simulink model "ScriptDemo"  (R2022b)
settings: configuration reference "TmVcThermal_Configuration_sub" (kept outside this file)
undefined symbols (not defined in the file): aaaa, bbbb, cTmComprCtrl_D_u8HvacFlowTable_db, cTmComprCtrl_D_u8HvacFlowTable_sw, cTmComprCtrl_n_i16ChillCmpIMax, cTmComprCtrl_n_i16ChillCmpIMin, cTmComprCtrl_n_i16ChillCmpIMin666, cTmComprCtrl_n_i16ChillCmpPMax, cTmComprCtrl_n_i16ChillCmpPMin, cTmComprCtrl_n_i16CmpChillCoolRpmKiMax, cTmComprCtrl_n_i16CmpChillCoolRpmKiMin, cTmComprCtrl_n_i16CmpChillCoolRpmKpMax, cTmComprCtrl_n_i16CmpChillCoolRpmKpMin, cTmComprCtrl_n_i16CmpCoolRpmKiMax, cTmComprCtrl_n_i16CmpCoolRpmKiMin, cTmComprCtrl_n_i16CmpCoolRpmKpMax, cTmComprCtrl_n_i16CmpCoolRpmKpMin, cTmComprCtrl_n_i16SM4CmpHeatKiMax, cTmComprCtrl_n_i16SM4CmpHeatKiMin, cTmComprCtrl_n_i16SM4CmpHeatKpMax, cTmComprCtrl_n_i16SM4CmpHeatKpMin, cTmComprCtrl_n_i16SM5CmpHeatKiMax, cTmComprCtrl_n_i16SM5CmpHeatKiMin, cTmComprCtrl_n_i16SM5CmpHeatKpMax, cTmComprCtrl_n_i16SM5CmpHeatKpMin, cTmComprCtrl_n_i16SM6CmpHeatKiMax, cTmComprCtrl_n_i16SM6CmpHeatKiMin, cTmComprCtrl_n_i16SM6CmpHeatKpMax, cTmComprCtrl_n_i16SM6CmpHeatKpMin, cTmComprCtrl_n_u16CmpMaxSpdFanFltLimt, cTmComprCtrl_n_u16CmpMaxSpdLoSidePFltLimt, cTmComprCtrl_n_u16CmpMaxSpdSensorFltLimt, cTmComprCtrl_n_u16CompMinRpm, cTmComprCtrl_n_u16CompRpmIncThres, cTmComprCtrl_t_u16BattCooltFFPeriod, cTmComprCtrl_t_u16BattCooltPIPeriod, cTmComprCtrl_t_u16CmpCoolFFPeriod, cTmComprCtrl_t_u16CmpCoolPIPeriod, cTmComprCtrl_t_u16CoolCmpChillFFPeriod, cTmComprCtrl_t_u16CoolCmpChillPIPeriod, cTmComprCtrl_t_u16SM4CmpHeatFFPeriod, cTmComprCtrl_t_u16SM4CmpHeatPIPeriod, cTmComprCtrl_t_u16SM5CmpHeatFFPeriod, cTmComprCtrl_t_u16SM5CmpHeatPIPeriod, cTmComprCtrl_t_u16SM6CmpHeatFFPeriod, cTmComprCtrl_t_u16SM6CmpHeatPIPeriod, cTmComprCtrl_Te_EvapClearInteg, cTmComprCtrl_Te_i16HpReqTempSaturoffset, cTmComprCtrl_Te_i16SatLpReplaceDiff, cTmComprCtrl_Te_i16SM3BatDiffStartEvapDecOffset, cTmComprCtrl_Te_i16SM3EvapLo, cTmComprCtrl_Te_i16SM3TBatDiffEntEvapDecOffset, cTmComprCtrl_Te_i16SM3TBatDiffEntEvapDecOffsetQuit, cTmComprCtrl_Te_s32ErrCmpChillPIContinueCoolH, cTmComprCtrl_Te_s32ErrCmpChillPIContinueCoolL, cTmComprCtrl_Te_s32ErrCmpPIContinueChillH, cTmComprCtrl_Te_s32ErrCmpPIContinueChillL, cTmComprCtrl_Te_s32ErrCmpPIContinueCoolH, cTmComprCtrl_Te_s32ErrCmpPIContinueCoolL, cTmComprCtrl_Te_s32ErrCmpPIContinueHeatH ... (+398)
libraries: simulink x782, PCMULib x640, simulink_need_slupdate x4
(part 33 of 41)

== system ScriptDemo/Create/createMerge/After/SM4/ID26297_SM4FF/Flow2Rpm/Subsystem4 ==
  In1 : Inport  OutDataTypeStr=int16
  Abs : Abs  OutDataTypeStr=uint16  SaturateOnIntegerOverflow=off
  Add6 : Sum  Inputs=+-  OutDataTypeStr=int16
  Compare To Constant : simulink/Logic and Bit Operations/Compare To Constant  relop=>=  const=0  OutDataTypeStr=boolean
  Compare To Constant1 : simulink/Logic and Bit Operations/Compare To Constant  relop=<=  const=10  OutDataTypeStr=boolean
  Constant6 : Constant  Value=0  OutDataTypeStr=uint16
  Constant7 : Constant  Value=10  OutDataTypeStr=uint16
  Logical Operator : Logic  AllPortsSameDT=off  OutDataTypeStr=boolean
  Switch : Switch  Criteria=u2 ~= 0  SaturateOnIntegerOverflow=off  InputSameDT=off
  Out1 : Outport
  wires:
  Add6/1 -> Switch/1
  Logical Operator/1 -> Switch/2
  Constant6/1 -> Switch/3
  Abs/1 -> Add6/2, Compare To Constant/1, Compare To Constant1/1
  Constant7/1 -> Add6/1
  Switch/1 -> Out1/1
  Compare To Constant1/1 -> Logical Operator/2
  Compare To Constant/1 -> Logical Operator/1
  In1/1 -> Abs/1

== system ScriptDemo/Create/createMerge/After/SM4/ID26297_SM4FF/Flow2Rpm/Subsystem5 ==
  In1 : Inport  OutDataTypeStr=int16
  Abs : Abs  OutDataTypeStr=uint16  SaturateOnIntegerOverflow=off
  Add6 : Sum  Inputs=+-  OutDataTypeStr=int16
  Compare To Constant : simulink/Logic and Bit Operations/Compare To Constant  relop=>=  const=0  OutDataTypeStr=boolean
  Compare To Constant1 : simulink/Logic and Bit Operations/Compare To Constant  relop=<=  const=10  OutDataTypeStr=boolean
  Constant6 : Constant  Value=0  OutDataTypeStr=uint16
  Constant7 : Constant  Value=10  OutDataTypeStr=uint16
  Logical Operator : Logic  AllPortsSameDT=off  OutDataTypeStr=boolean
  Switch : Switch  Criteria=u2 ~= 0  SaturateOnIntegerOverflow=off  InputSameDT=off
  Out1 : Outport
  wires:
  Add6/1 -> Switch/1
  Logical Operator/1 -> Switch/2
  Constant6/1 -> Switch/3
  Abs/1 -> Add6/2, Compare To Constant/1, Compare To Constant1/1
  Constant7/1 -> Add6/1
  Switch/1 -> Out1/1
  Compare To Constant1/1 -> Logical Operator/2
  Compare To Constant/1 -> Logical Operator/1
  In1/1 -> Abs/1

== system ScriptDemo/Create/createMerge/After/SM4/ID26297_SM4FF/Flow2Rpm/XCP ==
  md_u8Blw : Inport
  Constant1 : Constant  Value=BlwHeatLevel_db
      settings: AttributesFormatString=%<Value>
  Constant28 : Constant  Value=BlwHeatLevel_sw
      settings: AttributesFormatString=%<Value>
  Switch : Switch  Criteria=u2 ~= 0  SaturateOnIntegerOverflow=off  InputSameDT=off
  Out1 : Outport
  wires:
  md_u8Blw/1 -> Switch/3
  Switch/1 -> Out1/1
  Constant28/1 -> Switch/2
  Constant1/1 -> Switch/1

== system ScriptDemo/Create/createMerge/After/SM4/SM4_Ki/Flow2Rpm/Subsystem1 ==
  In1 : Inport  OutDataTypeStr=int16
  Abs : Abs  OutDataTypeStr=single  SaturateOnIntegerOverflow=off
  Add6 : Sum  Inputs=+-  OutDataTypeStr=int16
  Compare To Constant : simulink/Logic and Bit Operations/Compare To Constant  relop=>=  const=0  OutDataTypeStr=boolean
  Compare To Constant1 : simulink/Logic and Bit Operations/Compare To Constant  relop=<=  const=10  OutDataTypeStr=boolean
  Constant6 : Constant  Value=0  OutDataTypeStr=uint16
  Constant7 : Constant  Value=10  OutDataTypeStr=uint16
  Logical Operator : Logic  AllPortsSameDT=off  OutDataTypeStr=boolean
  Switch : Switch  Criteria=u2 ~= 0  SaturateOnIntegerOverflow=off  InputSameDT=off
  Out1 : Outport
  wires:
  Add6/1 -> Switch/1
  Logical Operator/1 -> Switch/2
  Constant6/1 -> Switch/3
  Abs/1 -> Add6/2, Compare To Constant/1, Compare To Constant1/1
  Constant7/1 -> Add6/1
  Switch/1 -> Out1/1
  Compare To Constant1/1 -> Logical Operator/2
  Compare To Constant/1 -> Logical Operator/1
  In1/1 -> Abs/1

== system ScriptDemo/Create/createMerge/After/SM4/SM4_Ki/Flow2Rpm/Subsystem2 ==
  In1 : Inport  OutDataTypeStr=int16
  Abs : Abs  OutDataTypeStr=uint16  SaturateOnIntegerOverflow=off
  Add6 : Sum  Inputs=+-  OutDataTypeStr=int16
  Compare To Constant : simulink/Logic and Bit Operations/Compare To Constant  relop=>=  const=0  OutDataTypeStr=boolean
  Compare To Constant1 : simulink/Logic and Bit Operations/Compare To Constant  relop=<=  const=10  OutDataTypeStr=boolean
  Constant6 : Constant  Value=0  OutDataTypeStr=uint16
  Constant7 : Constant  Value=10  OutDataTypeStr=uint16
  Logical Operator : Logic  AllPortsSameDT=off  OutDataTypeStr=boolean
  Switch : Switch  Criteria=u2 ~= 0  SaturateOnIntegerOverflow=off  InputSameDT=off
  Out1 : Outport
  wires:
  Add6/1 -> Switch/1
  Logical Operator/1 -> Switch/2
  Constant6/1 -> Switch/3
  Abs/1 -> Add6/2, Compare To Constant/1, Compare To Constant1/1
  Constant7/1 -> Add6/1
  Switch/1 -> Out1/1
  Compare To Constant1/1 -> Logical Operator/2
  Compare To Constant/1 -> Logical Operator/1
  In1/1 -> Abs/1

== system ScriptDemo/Create/createMerge/After/SM4/SM4_Ki/Flow2Rpm/Subsystem3 ==
  In1 : Inport  OutDataTypeStr=int16
  Abs : Abs  OutDataTypeStr=uint16  SaturateOnIntegerOverflow=off
  Add6 : Sum  Inputs=+-  OutDataTypeStr=int16
  Compare To Constant : simulink/Logic and Bit Operations/Compare To Constant  relop=>=  const=0  OutDataTypeStr=boolean
  Compare To Constant1 : simulink/Logic and Bit Operations/Compare To Constant  relop=<=  const=10  OutDataTypeStr=boolean
  Constant6 : Constant  Value=0  OutDataTypeStr=uint16
  Constant7 : Constant  Value=10  OutDataTypeStr=uint16
  Logical Operator : Logic  AllPortsSameDT=off  OutDataTypeStr=boolean
  Switch : Switch  Criteria=u2 ~= 0  SaturateOnIntegerOverflow=off  InputSameDT=off
  Out1 : Outport
  wires:
  Add6/1 -> Switch/1
  Logical Operator/1 -> Switch/2
  Constant6/1 -> Switch/3
  Abs/1 -> Add6/2, Compare To Constant/1, Compare To Constant1/1
  Constant7/1 -> Add6/1
  Switch/1 -> Out1/1
  Compare To Constant1/1 -> Logical Operator/2
  Compare To Constant/1 -> Logical Operator/1
  In1/1 -> Abs/1

== system ScriptDemo/Create/createMerge/After/SM4/SM4_Ki/Flow2Rpm/Subsystem4 ==
  In1 : Inport  OutDataTypeStr=int16
  Abs : Abs  OutDataTypeStr=uint16  SaturateOnIntegerOverflow=off
  Add6 : Sum  Inputs=+-  OutDataTypeStr=int16
  Compare To Constant : simulink/Logic and Bit Operations/Compare To Constant  relop=>=  const=0  OutDataTypeStr=boolean
  Compare To Constant1 : simulink/Logic and Bit Operations/Compare To Constant  relop=<=  const=10  OutDataTypeStr=boolean
  Constant6 : Constant  Value=0  OutDataTypeStr=uint16
  Constant7 : Constant  Value=10  OutDataTypeStr=uint16
  Logical Operator : Logic  AllPortsSameDT=off  OutDataTypeStr=boolean
  Switch : Switch  Criteria=u2 ~= 0  SaturateOnIntegerOverflow=off  InputSameDT=off
  Out1 : Outport
  wires:
  Add6/1 -> Switch/1
  Logical Operator/1 -> Switch/2
  Constant6/1 -> Switch/3
  Abs/1 -> Add6/2, Compare To Constant/1, Compare To Constant1/1
  Constant7/1 -> Add6/1
  Switch/1 -> Out1/1
  Compare To Constant1/1 -> Logical Operator/2
  Compare To Constant/1 -> Logical Operator/1
  In1/1 -> Abs/1

== system ScriptDemo/Create/createMerge/After/SM4/SM4_Ki/Flow2Rpm/Subsystem5 ==
  In1 : Inport  OutDataTypeStr=int16
  Abs : Abs  OutDataTypeStr=uint16  SaturateOnIntegerOverflow=off
  Add6 : Sum  Inputs=+-  OutDataTypeStr=int16
  Compare To Constant : simulink/Logic and Bit Operations/Compare To Constant  relop=>=  const=0  OutDataTypeStr=boolean
  Compare To Constant1 : simulink/Logic and Bit Operations/Compare To Constant  relop=<=  const=10  OutDataTypeStr=boolean
  Constant6 : Constant  Value=0  OutDataTypeStr=uint16
  Constant7 : Constant  Value=10  OutDataTypeStr=uint16
  Logical Operator : Logic  AllPortsSameDT=off  OutDataTypeStr=boolean
  Switch : Switch  Criteria=u2 ~= 0  SaturateOnIntegerOverflow=off  InputSameDT=off
  Out1 : Outport
  wires:
  Add6/1 -> Switch/1
  Logical Operator/1 -> Switch/2
  Constant6/1 -> Switch/3
  Abs/1 -> Add6/2, Compare To Constant/1, Compare To Constant1/1
  Constant7/1 -> Add6/1
  Switch/1 -> Out1/1
  Compare To Constant1/1 -> Logical Operator/2
  Compare To Constant/1 -> Logical Operator/1
  In1/1 -> Abs/1

== system ScriptDemo/Create/createMerge/After/SM4/SM4_Ki/Flow2Rpm/XCP ==
  md_u8Blw : Inport
  Constant1 : Constant  Value=BlwHeatLevel_db
      settings: AttributesFormatString=%<Value>
  Constant28 : Constant  Value=BlwHeatLevel_sw
      settings: AttributesFormatString=%<Value>
  Switch : Switch  Criteria=u2 ~= 0  SaturateOnIntegerOverflow=off  InputSameDT=off
  Out1 : Outport
  wires:
  md_u8Blw/1 -> Switch/3
  Switch/1 -> Out1/1
  Constant28/1 -> Switch/2
  Constant1/1 -> Switch/1

== system ScriptDemo/Create/createMerge/After/SM4/SM4_Kp/Flow2Rpm/Subsystem1 ==
  In1 : Inport  OutDataTypeStr=int16
  Abs : Abs  OutDataTypeStr=single  SaturateOnIntegerOverflow=off
  Add6 : Sum  Inputs=+-  OutDataTypeStr=int16
  Compare To Constant : simulink/Logic and Bit Operations/Compare To Constant  relop=>=  const=0  OutDataTypeStr=boolean
  Compare To Constant1 : simulink/Logic and Bit Operations/Compare To Constant  relop=<=  const=10  OutDataTypeStr=boolean
  Constant6 : Constant  Value=0  OutDataTypeStr=uint16
  Constant7 : Constant  Value=10  OutDataTypeStr=uint16
  Logical Operator : Logic  AllPortsSameDT=off  OutDataTypeStr=boolean
  Switch : Switch  Criteria=u2 ~= 0  SaturateOnIntegerOverflow=off  InputSameDT=off
  Out1 : Outport
  wires:
  Add6/1 -> Switch/1
  Logical Operator/1 -> Switch/2
  Constant6/1 -> Switch/3
  Abs/1 -> Add6/2, Compare To Constant/1, Compare To Constant1/1
  Constant7/1 -> Add6/1
  Switch/1 -> Out1/1
  Compare To Constant1/1 -> Logical Operator/2
  Compare To Constant/1 -> Logical Operator/1
  In1/1 -> Abs/1

== system ScriptDemo/Create/createMerge/After/SM4/SM4_Kp/Flow2Rpm/Subsystem2 ==
  In1 : Inport  OutDataTypeStr=int16
  Abs : Abs  OutDataTypeStr=uint16  SaturateOnIntegerOverflow=off
  Add6 : Sum  Inputs=+-  OutDataTypeStr=int16
  Compare To Constant : simulink/Logic and Bit Operations/Compare To Constant  relop=>=  const=0  OutDataTypeStr=boolean
  Compare To Constant1 : simulink/Logic and Bit Operations/Compare To Constant  relop=<=  const=10  OutDataTypeStr=boolean
  Constant6 : Constant  Value=0  OutDataTypeStr=uint16
  Constant7 : Constant  Value=10  OutDataTypeStr=uint16
  Logical Operator : Logic  AllPortsSameDT=off  OutDataTypeStr=boolean
  Switch : Switch  Criteria=u2 ~= 0  SaturateOnIntegerOverflow=off  InputSameDT=off
  Out1 : Outport
  wires:
  Add6/1 -> Switch/1
  Logical Operator/1 -> Switch/2
  Constant6/1 -> Switch/3
  Abs/1 -> Add6/2, Compare To Constant/1, Compare To Constant1/1
  Constant7/1 -> Add6/1
  Switch/1 -> Out1/1
  Compare To Constant1/1 -> Logical Operator/2
  Compare To Constant/1 -> Logical Operator/1
  In1/1 -> Abs/1

== system ScriptDemo/Create/createMerge/After/SM4/SM4_Kp/Flow2Rpm/Subsystem3 ==
  In1 : Inport  OutDataTypeStr=int16
  Abs : Abs  OutDataTypeStr=uint16  SaturateOnIntegerOverflow=off
  Add6 : Sum  Inputs=+-  OutDataTypeStr=int16
  Compare To Constant : simulink/Logic and Bit Operations/Compare To Constant  relop=>=  const=0  OutDataTypeStr=boolean
  Compare To Constant1 : simulink/Logic and Bit Operations/Compare To Constant  relop=<=  const=10  OutDataTypeStr=boolean
  Constant6 : Constant  Value=0  OutDataTypeStr=uint16
  Constant7 : Constant  Value=10  OutDataTypeStr=uint16
  Logical Operator : Logic  AllPortsSameDT=off  OutDataTypeStr=boolean
  Switch : Switch  Criteria=u2 ~= 0  SaturateOnIntegerOverflow=off  InputSameDT=off
  Out1 : Outport
  wires:
  Add6/1 -> Switch/1
  Logical Operator/1 -> Switch/2
  Constant6/1 -> Switch/3
  Abs/1 -> Add6/2, Compare To Constant/1, Compare To Constant1/1
  Constant7/1 -> Add6/1
  Switch/1 -> Out1/1
  Compare To Constant1/1 -> Logical Operator/2
  Compare To Constant/1 -> Logical Operator/1
  In1/1 -> Abs/1

== system ScriptDemo/Create/createMerge/After/SM4/SM4_Kp/Flow2Rpm/Subsystem4 ==
  In1 : Inport  OutDataTypeStr=int16
  Abs : Abs  OutDataTypeStr=uint16  SaturateOnIntegerOverflow=off
  Add6 : Sum  Inputs=+-  OutDataTypeStr=int16
  Compare To Constant : simulink/Logic and Bit Operations/Compare To Constant  relop=>=  const=0  OutDataTypeStr=boolean
  Compare To Constant1 : simulink/Logic and Bit Operations/Compare To Constant  relop=<=  const=10  OutDataTypeStr=boolean
  Constant6 : Constant  Value=0  OutDataTypeStr=uint16
  Constant7 : Constant  Value=10  OutDataTypeStr=uint16
  Logical Operator : Logic  AllPortsSameDT=off  OutDataTypeStr=boolean
  Switch : Switch  Criteria=u2 ~= 0  SaturateOnIntegerOverflow=off  InputSameDT=off
  Out1 : Outport
  wires:
  Add6/1 -> Switch/1
  Logical Operator/1 -> Switch/2
  Constant6/1 -> Switch/3
  Abs/1 -> Add6/2, Compare To Constant/1, Compare To Constant1/1
  Constant7/1 -> Add6/1
  Switch/1 -> Out1/1
  Compare To Constant1/1 -> Logical Operator/2
  Compare To Constant/1 -> Logical Operator/1
  In1/1 -> Abs/1

== system ScriptDemo/Create/createMerge/After/SM4/SM4_Kp/Flow2Rpm/Subsystem5 ==
  In1 : Inport  OutDataTypeStr=int16
  Abs : Abs  OutDataTypeStr=uint16  SaturateOnIntegerOverflow=off
  Add6 : Sum  Inputs=+-  OutDataTypeStr=int16
  Compare To Constant : simulink/Logic and Bit Operations/Compare To Constant  relop=>=  const=0  OutDataTypeStr=boolean
  Compare To Constant1 : simulink/Logic and Bit Operations/Compare To Constant  relop=<=  const=10  OutDataTypeStr=boolean
  Constant6 : Constant  Value=0  OutDataTypeStr=uint16
  Constant7 : Constant  Value=10  OutDataTypeStr=uint16
  Logical Operator : Logic  AllPortsSameDT=off  OutDataTypeStr=boolean
  Switch : Switch  Criteria=u2 ~= 0  SaturateOnIntegerOverflow=off  InputSameDT=off
  Out1 : Outport
  wires:
  Add6/1 -> Switch/1
  Logical Operator/1 -> Switch/2
  Constant6/1 -> Switch/3
  Abs/1 -> Add6/2, Compare To Constant/1, Compare To Constant1/1
  Constant7/1 -> Add6/1
  Switch/1 -> Out1/1
  Compare To Constant1/1 -> Logical Operator/2
  Compare To Constant/1 -> Logical Operator/1
  In1/1 -> Abs/1

== system ScriptDemo/Create/createMerge/After/SM4/SM4_Kp/Flow2Rpm/XCP ==
  md_u8Blw : Inport
  Constant1 : Constant  Value=BlwHeatLevel_db
      settings: AttributesFormatString=%<Value>
  Constant28 : Constant  Value=BlwHeatLevel_sw
      settings: AttributesFormatString=%<Value>
  Switch : Switch  Criteria=u2 ~= 0  SaturateOnIntegerOverflow=off  InputSameDT=off
  Out1 : Outport
  wires:
  md_u8Blw/1 -> Switch/3
  Switch/1 -> Out1/1
  Constant28/1 -> Switch/2
  Constant1/1 -> Switch/1

== system ScriptDemo/Create/createMerge/After/SM5/ID26291_SM5FF/Flow2Rpm/Subsystem1 ==
  In1 : Inport  OutDataTypeStr=int16
  Abs : Abs  OutDataTypeStr=single  SaturateOnIntegerOverflow=off
  Add6 : Sum  Inputs=+-  OutDataTypeStr=int16
  Compare To Constant : simulink/Logic and Bit Operations/Compare To Constant  relop=>=  const=0  OutDataTypeStr=boolean
  Compare To Constant1 : simulink/Logic and Bit Operations/Compare To Constant  relop=<=  const=10  OutDataTypeStr=boolean
  Constant6 : Constant  Value=0  OutDataTypeStr=uint16
  Constant7 : Constant  Value=10  OutDataTypeStr=uint16
  Logical Operator : Logic  AllPortsSameDT=off  OutDataTypeStr=boolean
  Switch : Switch  Criteria=u2 ~= 0  SaturateOnIntegerOverflow=off  InputSameDT=off
  Out1 : Outport
  wires:
  Add6/1 -> Switch/1
  Logical Operator/1 -> Switch/2
  Constant6/1 -> Switch/3
  Abs/1 -> Add6/2, Compare To Constant/1, Compare To Constant1/1
  Constant7/1 -> Add6/1
  Switch/1 -> Out1/1
  Compare To Constant1/1 -> Logical Operator/2
  Compare To Constant/1 -> Logical Operator/1
  In1/1 -> Abs/1

== system ScriptDemo/Create/createMerge/After/SM5/ID26291_SM5FF/Flow2Rpm/Subsystem2 ==
  In1 : Inport  OutDataTypeStr=int16
  Abs : Abs  OutDataTypeStr=uint16  SaturateOnIntegerOverflow=off
  Add6 : Sum  Inputs=+-  OutDataTypeStr=int16
  Compare To Constant : simulink/Logic and Bit Operations/Compare To Constant  relop=>=  const=0  OutDataTypeStr=boolean
  Compare To Constant1 : simulink/Logic and Bit Operations/Compare To Constant  relop=<=  const=10  OutDataTypeStr=boolean
  Constant6 : Constant  Value=0  OutDataTypeStr=uint16
  Constant7 : Constant  Value=10  OutDataTypeStr=uint16
  Logical Operator : Logic  AllPortsSameDT=off  OutDataTypeStr=boolean
  Switch : Switch  Criteria=u2 ~= 0  SaturateOnIntegerOverflow=off  InputSameDT=off
  Out1 : Outport
  wires:
  Add6/1 -> Switch/1
  Logical Operator/1 -> Switch/2
  Constant6/1 -> Switch/3
  Abs/1 -> Add6/2, Compare To Constant/1, Compare To Constant1/1
  Constant7/1 -> Add6/1
  Switch/1 -> Out1/1
  Compare To Constant1/1 -> Logical Operator/2
  Compare To Constant/1 -> Logical Operator/1
  In1/1 -> Abs/1

== system ScriptDemo/Create/createMerge/After/SM5/ID26291_SM5FF/Flow2Rpm/Subsystem3 ==
  In1 : Inport  OutDataTypeStr=int16
  Abs : Abs  OutDataTypeStr=uint16  SaturateOnIntegerOverflow=off
  Add6 : Sum  Inputs=+-  OutDataTypeStr=int16
  Compare To Constant : simulink/Logic and Bit Operations/Compare To Constant  relop=>=  const=0  OutDataTypeStr=boolean
  Compare To Constant1 : simulink/Logic and Bit Operations/Compare To Constant  relop=<=  const=10  OutDataTypeStr=boolean
  Constant6 : Constant  Value=0  OutDataTypeStr=uint16
  Constant7 : Constant  Value=10  OutDataTypeStr=uint16
  Logical Operator : Logic  AllPortsSameDT=off  OutDataTypeStr=boolean
  Switch : Switch  Criteria=u2 ~= 0  SaturateOnIntegerOverflow=off  InputSameDT=off
  Out1 : Outport
  wires:
  Add6/1 -> Switch/1
  Logical Operator/1 -> Switch/2
  Constant6/1 -> Switch/3
  Abs/1 -> Add6/2, Compare To Constant/1, Compare To Constant1/1
  Constant7/1 -> Add6/1
  Switch/1 -> Out1/1
  Compare To Constant1/1 -> Logical Operator/2
  Compare To Constant/1 -> Logical Operator/1
  In1/1 -> Abs/1

== system ScriptDemo/Create/createMerge/After/SM5/ID26291_SM5FF/Flow2Rpm/Subsystem4 ==
  In1 : Inport  OutDataTypeStr=int16
  Abs : Abs  OutDataTypeStr=uint16  SaturateOnIntegerOverflow=off
  Add6 : Sum  Inputs=+-  OutDataTypeStr=int16
  Compare To Constant : simulink/Logic and Bit Operations/Compare To Constant  relop=>=  const=0  OutDataTypeStr=boolean
  Compare To Constant1 : simulink/Logic and Bit Operations/Compare To Constant  relop=<=  const=10  OutDataTypeStr=boolean
  Constant6 : Constant  Value=0  OutDataTypeStr=uint16
  Constant7 : Constant  Value=10  OutDataTypeStr=uint16
  Logical Operator : Logic  AllPortsSameDT=off  OutDataTypeStr=boolean
  Switch : Switch  Criteria=u2 ~= 0  SaturateOnIntegerOverflow=off  InputSameDT=off
  Out1 : Outport
  wires:
  Add6/1 -> Switch/1
  Logical Operator/1 -> Switch/2
  Constant6/1 -> Switch/3
  Abs/1 -> Add6/2, Compare To Constant/1, Compare To Constant1/1
  Constant7/1 -> Add6/1
  Switch/1 -> Out1/1
  Compare To Constant1/1 -> Logical Operator/2
  Compare To Constant/1 -> Logical Operator/1
  In1/1 -> Abs/1

== system ScriptDemo/Create/createMerge/After/SM5/ID26291_SM5FF/Flow2Rpm/Subsystem5 ==
  In1 : Inport  OutDataTypeStr=int16
  Abs : Abs  OutDataTypeStr=uint16  SaturateOnIntegerOverflow=off
  Add6 : Sum  Inputs=+-  OutDataTypeStr=int16
  Compare To Constant : simulink/Logic and Bit Operations/Compare To Constant  relop=>=  const=0  OutDataTypeStr=boolean
  Compare To Constant1 : simulink/Logic and Bit Operations/Compare To Constant  relop=<=  const=10  OutDataTypeStr=boolean
  Constant6 : Constant  Value=0  OutDataTypeStr=uint16
  Constant7 : Constant  Value=10  OutDataTypeStr=uint16
  Logical Operator : Logic  AllPortsSameDT=off  OutDataTypeStr=boolean
  Switch : Switch  Criteria=u2 ~= 0  SaturateOnIntegerOverflow=off  InputSameDT=off
  Out1 : Outport
  wires:
  Add6/1 -> Switch/1
  Logical Operator/1 -> Switch/2
  Constant6/1 -> Switch/3
  Abs/1 -> Add6/2, Compare To Constant/1, Compare To Constant1/1
  Constant7/1 -> Add6/1
  Switch/1 -> Out1/1
  Compare To Constant1/1 -> Logical Operator/2
  Compare To Constant/1 -> Logical Operator/1
  In1/1 -> Abs/1

== system ScriptDemo/Create/createMerge/After/SM5/ID26291_SM5FF/Flow2Rpm/XCP ==
  md_u8Blw : Inport
  Constant1 : Constant  Value=BlwHeatLevel_db
      settings: AttributesFormatString=%<Value>
  Constant28 : Constant  Value=BlwHeatLevel_sw
      settings: AttributesFormatString=%<Value>
  Switch : Switch  Criteria=u2 ~= 0  SaturateOnIntegerOverflow=off  InputSameDT=off
  Out1 : Outport
  wires:
  md_u8Blw/1 -> Switch/3
  Switch/1 -> Out1/1
  Constant28/1 -> Switch/2
  Constant1/1 -> Switch/1

== system ScriptDemo/Create/createMerge/After/SM5/SM5_Ki/Flow2Rpm/Subsystem1 ==
  In1 : Inport  OutDataTypeStr=int16
  Abs : Abs  OutDataTypeStr=single  SaturateOnIntegerOverflow=off
  Add6 : Sum  Inputs=+-  OutDataTypeStr=int16
  Compare To Constant : simulink/Logic and Bit Operations/Compare To Constant  relop=>=  const=0  OutDataTypeStr=boolean
  Compare To Constant1 : simulink/Logic and Bit Operations/Compare To Constant  relop=<=  const=10  OutDataTypeStr=boolean
  Constant6 : Constant  Value=0  OutDataTypeStr=uint16
  Constant7 : Constant  Value=10  OutDataTypeStr=uint16
  Logical Operator : Logic  AllPortsSameDT=off  OutDataTypeStr=boolean
  Switch : Switch  Criteria=u2 ~= 0  SaturateOnIntegerOverflow=off  InputSameDT=off
  Out1 : Outport
  wires:
  Add6/1 -> Switch/1
  Logical Operator/1 -> Switch/2
  Constant6/1 -> Switch/3
  Abs/1 -> Add6/2, Compare To Constant/1, Compare To Constant1/1
  Constant7/1 -> Add6/1
  Switch/1 -> Out1/1
  Compare To Constant1/1 -> Logical Operator/2
  Compare To Constant/1 -> Logical Operator/1
  In1/1 -> Abs/1

== system ScriptDemo/Create/createMerge/After/SM5/SM5_Ki/Flow2Rpm/Subsystem2 ==
  In1 : Inport  OutDataTypeStr=int16
  Abs : Abs  OutDataTypeStr=uint16  SaturateOnIntegerOverflow=off
  Add6 : Sum  Inputs=+-  OutDataTypeStr=int16
  Compare To Constant : simulink/Logic and Bit Operations/Compare To Constant  relop=>=  const=0  OutDataTypeStr=boolean
  Compare To Constant1 : simulink/Logic and Bit Operations/Compare To Constant  relop=<=  const=10  OutDataTypeStr=boolean
  Constant6 : Constant  Value=0  OutDataTypeStr=uint16
  Constant7 : Constant  Value=10  OutDataTypeStr=uint16
  Logical Operator : Logic  AllPortsSameDT=off  OutDataTypeStr=boolean
  Switch : Switch  Criteria=u2 ~= 0  SaturateOnIntegerOverflow=off  InputSameDT=off
  Out1 : Outport
  wires:
  Add6/1 -> Switch/1
  Logical Operator/1 -> Switch/2
  Constant6/1 -> Switch/3
  Abs/1 -> Add6/2, Compare To Constant/1, Compare To Constant1/1
  Constant7/1 -> Add6/1
  Switch/1 -> Out1/1
  Compare To Constant1/1 -> Logical Operator/2
  Compare To Constant/1 -> Logical Operator/1
  In1/1 -> Abs/1

== system ScriptDemo/Create/createMerge/After/SM5/SM5_Ki/Flow2Rpm/Subsystem3 ==
  In1 : Inport  OutDataTypeStr=int16
  Abs : Abs  OutDataTypeStr=uint16  SaturateOnIntegerOverflow=off
  Add6 : Sum  Inputs=+-  OutDataTypeStr=int16
  Compare To Constant : simulink/Logic and Bit Operations/Compare To Constant  relop=>=  const=0  OutDataTypeStr=boolean
  Compare To Constant1 : simulink/Logic and Bit Operations/Compare To Constant  relop=<=  const=10  OutDataTypeStr=boolean
  Constant6 : Constant  Value=0  OutDataTypeStr=uint16
  Constant7 : Constant  Value=10  OutDataTypeStr=uint16
  Logical Operator : Logic  AllPortsSameDT=off  OutDataTypeStr=boolean
  Switch : Switch  Criteria=u2 ~= 0  SaturateOnIntegerOverflow=off  InputSameDT=off
  Out1 : Outport
  wires:
  Add6/1 -> Switch/1
  Logical Operator/1 -> Switch/2
  Constant6/1 -> Switch/3
  Abs/1 -> Add6/2, Compare To Constant/1, Compare To Constant1/1
  Constant7/1 -> Add6/1
  Switch/1 -> Out1/1
  Compare To Constant1/1 -> Logical Operator/2
  Compare To Constant/1 -> Logical Operator/1
  In1/1 -> Abs/1

== system ScriptDemo/Create/createMerge/After/SM5/SM5_Ki/Flow2Rpm/Subsystem4 ==
  In1 : Inport  OutDataTypeStr=int16
  Abs : Abs  OutDataTypeStr=uint16  SaturateOnIntegerOverflow=off
  Add6 : Sum  Inputs=+-  OutDataTypeStr=int16
  Compare To Constant : simulink/Logic and Bit Operations/Compare To Constant  relop=>=  const=0  OutDataTypeStr=boolean
  Compare To Constant1 : simulink/Logic and Bit Operations/Compare To Constant  relop=<=  const=10  OutDataTypeStr=boolean
  Constant6 : Constant  Value=0  OutDataTypeStr=uint16
  Constant7 : Constant  Value=10  OutDataTypeStr=uint16
  Logical Operator : Logic  AllPortsSameDT=off  OutDataTypeStr=boolean
  Switch : Switch  Criteria=u2 ~= 0  SaturateOnIntegerOverflow=off  InputSameDT=off
  Out1 : Outport
  wires:
  Add6/1 -> Switch/1
  Logical Operator/1 -> Switch/2
  Constant6/1 -> Switch/3
  Abs/1 -> Add6/2, Compare To Constant/1, Compare To Constant1/1
  Constant7/1 -> Add6/1
  Switch/1 -> Out1/1
  Compare To Constant1/1 -> Logical Operator/2
  Compare To Constant/1 -> Logical Operator/1
  In1/1 -> Abs/1

== system ScriptDemo/Create/createMerge/After/SM5/SM5_Ki/Flow2Rpm/Subsystem5 ==
  In1 : Inport  OutDataTypeStr=int16
  Abs : Abs  OutDataTypeStr=uint16  SaturateOnIntegerOverflow=off
  Add6 : Sum  Inputs=+-  OutDataTypeStr=int16
  Compare To Constant : simulink/Logic and Bit Operations/Compare To Constant  relop=>=  const=0  OutDataTypeStr=boolean
  Compare To Constant1 : simulink/Logic and Bit Operations/Compare To Constant  relop=<=  const=10  OutDataTypeStr=boolean
  Constant6 : Constant  Value=0  OutDataTypeStr=uint16
  Constant7 : Constant  Value=10  OutDataTypeStr=uint16
  Logical Operator : Logic  AllPortsSameDT=off  OutDataTypeStr=boolean
  Switch : Switch  Criteria=u2 ~= 0  SaturateOnIntegerOverflow=off  InputSameDT=off
  Out1 : Outport
  wires:
  Add6/1 -> Switch/1
  Logical Operator/1 -> Switch/2
  Constant6/1 -> Switch/3
  Abs/1 -> Add6/2, Compare To Constant/1, Compare To Constant1/1
  Constant7/1 -> Add6/1
  Switch/1 -> Out1/1
  Compare To Constant1/1 -> Logical Operator/2
  Compare To Constant/1 -> Logical Operator/1
  In1/1 -> Abs/1

== system ScriptDemo/Create/createMerge/After/SM5/SM5_Ki/Flow2Rpm/XCP ==
  md_u8Blw : Inport
  Constant1 : Constant  Value=BlwHeatLevel_db
      settings: AttributesFormatString=%<Value>
  Constant28 : Constant  Value=BlwHeatLevel_sw
      settings: AttributesFormatString=%<Value>
  Switch : Switch  Criteria=u2 ~= 0  SaturateOnIntegerOverflow=off  InputSameDT=off
  Out1 : Outport
  wires:
  md_u8Blw/1 -> Switch/3
  Switch/1 -> Out1/1
  Constant28/1 -> Switch/2
  Constant1/1 -> Switch/1

== system ScriptDemo/Create/createMerge/After/SM5/SM5_Kp/Flow2Rpm/Subsystem1 ==
  In1 : Inport  OutDataTypeStr=int16
  Abs : Abs  OutDataTypeStr=single  SaturateOnIntegerOverflow=off
  Add6 : Sum  Inputs=+-  OutDataTypeStr=int16
  Compare To Constant : simulink/Logic and Bit Operations/Compare To Constant  relop=>=  const=0  OutDataTypeStr=boolean
  Compare To Constant1 : simulink/Logic and Bit Operations/Compare To Constant  relop=<=  const=10  OutDataTypeStr=boolean
  Constant6 : Constant  Value=0  OutDataTypeStr=uint16
  Constant7 : Constant  Value=10  OutDataTypeStr=uint16
  Logical Operator : Logic  AllPortsSameDT=off  OutDataTypeStr=boolean
  Switch : Switch  Criteria=u2 ~= 0  SaturateOnIntegerOverflow=off  InputSameDT=off
  Out1 : Outport
  wires:
  Add6/1 -> Switch/1
  Logical Operator/1 -> Switch/2
  Constant6/1 -> Switch/3
  Abs/1 -> Add6/2, Compare To Constant/1, Compare To Constant1/1
  Constant7/1 -> Add6/1
  Switch/1 -> Out1/1
  Compare To Constant1/1 -> Logical Operator/2
  Compare To Constant/1 -> Logical Operator/1
  In1/1 -> Abs/1

== system ScriptDemo/Create/createMerge/After/SM5/SM5_Kp/Flow2Rpm/Subsystem2 ==
  In1 : Inport  OutDataTypeStr=int16
  Abs : Abs  OutDataTypeStr=uint16  SaturateOnIntegerOverflow=off
  Add6 : Sum  Inputs=+-  OutDataTypeStr=int16
  Compare To Constant : simulink/Logic and Bit Operations/Compare To Constant  relop=>=  const=0  OutDataTypeStr=boolean
  Compare To Constant1 : simulink/Logic and Bit Operations/Compare To Constant  relop=<=  const=10  OutDataTypeStr=boolean
  Constant6 : Constant  Value=0  OutDataTypeStr=uint16
  Constant7 : Constant  Value=10  OutDataTypeStr=uint16
  Logical Operator : Logic  AllPortsSameDT=off  OutDataTypeStr=boolean
  Switch : Switch  Criteria=u2 ~= 0  SaturateOnIntegerOverflow=off  InputSameDT=off
  Out1 : Outport
  wires:
  Add6/1 -> Switch/1
  Logical Operator/1 -> Switch/2
  Constant6/1 -> Switch/3
  Abs/1 -> Add6/2, Compare To Constant/1, Compare To Constant1/1
  Constant7/1 -> Add6/1
  Switch/1 -> Out1/1
  Compare To Constant1/1 -> Logical Operator/2
  Compare To Constant/1 -> Logical Operator/1
  In1/1 -> Abs/1

== system ScriptDemo/Create/createMerge/After/SM5/SM5_Kp/Flow2Rpm/Subsystem3 ==
  In1 : Inport  OutDataTypeStr=int16
  Abs : Abs  OutDataTypeStr=uint16  SaturateOnIntegerOverflow=off
  Add6 : Sum  Inputs=+-  OutDataTypeStr=int16
  Compare To Constant : simulink/Logic and Bit Operations/Compare To Constant  relop=>=  const=0  OutDataTypeStr=boolean
  Compare To Constant1 : simulink/Logic and Bit Operations/Compare To Constant  relop=<=  const=10  OutDataTypeStr=boolean
  Constant6 : Constant  Value=0  OutDataTypeStr=uint16
  Constant7 : Constant  Value=10  OutDataTypeStr=uint16
  Logical Operator : Logic  AllPortsSameDT=off  OutDataTypeStr=boolean
  Switch : Switch  Criteria=u2 ~= 0  SaturateOnIntegerOverflow=off  InputSameDT=off
  Out1 : Outport
  wires:
  Add6/1 -> Switch/1
  Logical Operator/1 -> Switch/2
  Constant6/1 -> Switch/3
  Abs/1 -> Add6/2, Compare To Constant/1, Compare To Constant1/1
  Constant7/1 -> Add6/1
  Switch/1 -> Out1/1
  Compare To Constant1/1 -> Logical Operator/2
  Compare To Constant/1 -> Logical Operator/1
  In1/1 -> Abs/1

== system ScriptDemo/Create/createMerge/After/SM5/SM5_Kp/Flow2Rpm/Subsystem4 ==
  In1 : Inport  OutDataTypeStr=int16
  Abs : Abs  OutDataTypeStr=uint16  SaturateOnIntegerOverflow=off
  Add6 : Sum  Inputs=+-  OutDataTypeStr=int16
  Compare To Constant : simulink/Logic and Bit Operations/Compare To Constant  relop=>=  const=0  OutDataTypeStr=boolean
  Compare To Constant1 : simulink/Logic and Bit Operations/Compare To Constant  relop=<=  const=10  OutDataTypeStr=boolean
  Constant6 : Constant  Value=0  OutDataTypeStr=uint16
  Constant7 : Constant  Value=10  OutDataTypeStr=uint16
  Logical Operator : Logic  AllPortsSameDT=off  OutDataTypeStr=boolean
  Switch : Switch  Criteria=u2 ~= 0  SaturateOnIntegerOverflow=off  InputSameDT=off
  Out1 : Outport
  wires:
  Add6/1 -> Switch/1
  Logical Operator/1 -> Switch/2
  Constant6/1 -> Switch/3
  Abs/1 -> Add6/2, Compare To Constant/1, Compare To Constant1/1
  Constant7/1 -> Add6/1
  Switch/1 -> Out1/1
  Compare To Constant1/1 -> Logical Operator/2
  Compare To Constant/1 -> Logical Operator/1
  In1/1 -> Abs/1

== system ScriptDemo/Create/createMerge/After/SM5/SM5_Kp/Flow2Rpm/Subsystem5 ==
  In1 : Inport  OutDataTypeStr=int16
  Abs : Abs  OutDataTypeStr=uint16  SaturateOnIntegerOverflow=off
  Add6 : Sum  Inputs=+-  OutDataTypeStr=int16
  Compare To Constant : simulink/Logic and Bit Operations/Compare To Constant  relop=>=  const=0  OutDataTypeStr=boolean
  Compare To Constant1 : simulink/Logic and Bit Operations/Compare To Constant  relop=<=  const=10  OutDataTypeStr=boolean
  Constant6 : Constant  Value=0  OutDataTypeStr=uint16
  Constant7 : Constant  Value=10  OutDataTypeStr=uint16
  Logical Operator : Logic  AllPortsSameDT=off  OutDataTypeStr=boolean
  Switch : Switch  Criteria=u2 ~= 0  SaturateOnIntegerOverflow=off  InputSameDT=off
  Out1 : Outport
  wires:
  Add6/1 -> Switch/1
  Logical Operator/1 -> Switch/2
  Constant6/1 -> Switch/3
  Abs/1 -> Add6/2, Compare To Constant/1, Compare To Constant1/1
  Constant7/1 -> Add6/1
  Switch/1 -> Out1/1
  Compare To Constant1/1 -> Logical Operator/2
  Compare To Constant/1 -> Logical Operator/1
  In1/1 -> Abs/1

== system ScriptDemo/Create/createMerge/After/SM5/SM5_Kp/Flow2Rpm/XCP ==
  md_u8Blw : Inport
  Constant1 : Constant  Value=BlwHeatLevel_db
      settings: AttributesFormatString=%<Value>
  Constant28 : Constant  Value=BlwHeatLevel_sw
      settings: AttributesFormatString=%<Value>
  Switch : Switch  Criteria=u2 ~= 0  SaturateOnIntegerOverflow=off  InputSameDT=off
  Out1 : Outport
  wires:
  md_u8Blw/1 -> Switch/3
  Switch/1 -> Out1/1
  Constant28/1 -> Switch/2
  Constant1/1 -> Switch/1

== system ScriptDemo/Create/createMerge/After/SM6/ID26282_SM6FF/Flow2Rpm/Subsystem1 ==
  In1 : Inport  OutDataTypeStr=int16
  Abs : Abs  OutDataTypeStr=single  SaturateOnIntegerOverflow=off
  Add6 : Sum  Inputs=+-  OutDataTypeStr=int16
  Compare To Constant : simulink/Logic and Bit Operations/Compare To Constant  relop=>=  const=0  OutDataTypeStr=boolean
  Compare To Constant1 : simulink/Logic and Bit Operations/Compare To Constant  relop=<=  const=10  OutDataTypeStr=boolean
  Constant6 : Constant  Value=0  OutDataTypeStr=uint16
  Constant7 : Constant  Value=10  OutDataTypeStr=uint16
  Logical Operator : Logic  AllPortsSameDT=off  OutDataTypeStr=boolean
  Switch : Switch  Criteria=u2 ~= 0  SaturateOnIntegerOverflow=off  InputSameDT=off
  Out1 : Outport
  wires:
  Add6/1 -> Switch/1
  Logical Operator/1 -> Switch/2
  Constant6/1 -> Switch/3
  Abs/1 -> Add6/2, Compare To Constant/1, Compare To Constant1/1
  Constant7/1 -> Add6/1
  Switch/1 -> Out1/1
  Compare To Constant1/1 -> Logical Operator/2
  Compare To Constant/1 -> Logical Operator/1
  In1/1 -> Abs/1

== system ScriptDemo/Create/createMerge/After/SM6/ID26282_SM6FF/Flow2Rpm/Subsystem2 ==
  In1 : Inport  OutDataTypeStr=int16
  Abs : Abs  OutDataTypeStr=uint16  SaturateOnIntegerOverflow=off
  Add6 : Sum  Inputs=+-  OutDataTypeStr=int16
  Compare To Constant : simulink/Logic and Bit Operations/Compare To Constant  relop=>=  const=0  OutDataTypeStr=boolean
  Compare To Constant1 : simulink/Logic and Bit Operations/Compare To Constant  relop=<=  const=10  OutDataTypeStr=boolean
  Constant6 : Constant  Value=0  OutDataTypeStr=uint16
  Constant7 : Constant  Value=10  OutDataTypeStr=uint16
  Logical Operator : Logic  AllPortsSameDT=off  OutDataTypeStr=boolean
  Switch : Switch  Criteria=u2 ~= 0  SaturateOnIntegerOverflow=off  InputSameDT=off
  Out1 : Outport
  wires:
  Add6/1 -> Switch/1
  Logical Operator/1 -> Switch/2
  Constant6/1 -> Switch/3
  Abs/1 -> Add6/2, Compare To Constant/1, Compare To Constant1/1
  Constant7/1 -> Add6/1
  Switch/1 -> Out1/1
  Compare To Constant1/1 -> Logical Operator/2
  Compare To Constant/1 -> Logical Operator/1
  In1/1 -> Abs/1

== system ScriptDemo/Create/createMerge/After/SM6/ID26282_SM6FF/Flow2Rpm/Subsystem3 ==
  In1 : Inport  OutDataTypeStr=int16
  Abs : Abs  OutDataTypeStr=uint16  SaturateOnIntegerOverflow=off
  Add6 : Sum  Inputs=+-  OutDataTypeStr=int16
  Compare To Constant : simulink/Logic and Bit Operations/Compare To Constant  relop=>=  const=0  OutDataTypeStr=boolean
  Compare To Constant1 : simulink/Logic and Bit Operations/Compare To Constant  relop=<=  const=10  OutDataTypeStr=boolean
  Constant6 : Constant  Value=0  OutDataTypeStr=uint16
  Constant7 : Constant  Value=10  OutDataTypeStr=uint16
  Logical Operator : Logic  AllPortsSameDT=off  OutDataTypeStr=boolean
  Switch : Switch  Criteria=u2 ~= 0  SaturateOnIntegerOverflow=off  InputSameDT=off
  Out1 : Outport
  wires:
  Add6/1 -> Switch/1
  Logical Operator/1 -> Switch/2
  Constant6/1 -> Switch/3
  Abs/1 -> Add6/2, Compare To Constant/1, Compare To Constant1/1
  Constant7/1 -> Add6/1
  Switch/1 -> Out1/1
  Compare To Constant1/1 -> Logical Operator/2
  Compare To Constant/1 -> Logical Operator/1
  In1/1 -> Abs/1

== system ScriptDemo/Create/createMerge/After/SM6/ID26282_SM6FF/Flow2Rpm/Subsystem4 ==
  In1 : Inport  OutDataTypeStr=int16
  Abs : Abs  OutDataTypeStr=uint16  SaturateOnIntegerOverflow=off
  Add6 : Sum  Inputs=+-  OutDataTypeStr=int16
  Compare To Constant : simulink/Logic and Bit Operations/Compare To Constant  relop=>=  const=0  OutDataTypeStr=boolean
  Compare To Constant1 : simulink/Logic and Bit Operations/Compare To Constant  relop=<=  const=10  OutDataTypeStr=boolean
  Constant6 : Constant  Value=0  OutDataTypeStr=uint16
  Constant7 : Constant  Value=10  OutDataTypeStr=uint16
  Logical Operator : Logic  AllPortsSameDT=off  OutDataTypeStr=boolean
  Switch : Switch  Criteria=u2 ~= 0  SaturateOnIntegerOverflow=off  InputSameDT=off
  Out1 : Outport
  wires:
  Add6/1 -> Switch/1
  Logical Operator/1 -> Switch/2
  Constant6/1 -> Switch/3
  Abs/1 -> Add6/2, Compare To Constant/1, Compare To Constant1/1
  Constant7/1 -> Add6/1
  Switch/1 -> Out1/1
  Compare To Constant1/1 -> Logical Operator/2
  Compare To Constant/1 -> Logical Operator/1
  In1/1 -> Abs/1

== system ScriptDemo/Create/createMerge/After/SM6/ID26282_SM6FF/Flow2Rpm/Subsystem5 ==
  In1 : Inport  OutDataTypeStr=int16
  Abs : Abs  OutDataTypeStr=uint16  SaturateOnIntegerOverflow=off
  Add6 : Sum  Inputs=+-  OutDataTypeStr=int16
  Compare To Constant : simulink/Logic and Bit Operations/Compare To Constant  relop=>=  const=0  OutDataTypeStr=boolean
  Compare To Constant1 : simulink/Logic and Bit Operations/Compare To Constant  relop=<=  const=10  OutDataTypeStr=boolean
  Constant6 : Constant  Value=0  OutDataTypeStr=uint16
  Constant7 : Constant  Value=10  OutDataTypeStr=uint16
  Logical Operator : Logic  AllPortsSameDT=off  OutDataTypeStr=boolean
  Switch : Switch  Criteria=u2 ~= 0  SaturateOnIntegerOverflow=off  InputSameDT=off
  Out1 : Outport
  wires:
  Add6/1 -> Switch/1
  Logical Operator/1 -> Switch/2
  Constant6/1 -> Switch/3
  Abs/1 -> Add6/2, Compare To Constant/1, Compare To Constant1/1
  Constant7/1 -> Add6/1
  Switch/1 -> Out1/1
  Compare To Constant1/1 -> Logical Operator/2
  Compare To Constant/1 -> Logical Operator/1
  In1/1 -> Abs/1

== system ScriptDemo/Create/createMerge/After/SM6/ID26282_SM6FF/Flow2Rpm/XCP ==
  md_u8Blw : Inport
  Constant1 : Constant  Value=BlwHeatLevel_db
      settings: AttributesFormatString=%<Value>
  Constant28 : Constant  Value=BlwHeatLevel_sw
      settings: AttributesFormatString=%<Value>
  Switch : Switch  Criteria=u2 ~= 0  SaturateOnIntegerOverflow=off  InputSameDT=off
  Out1 : Outport
  wires:
  md_u8Blw/1 -> Switch/3
  Switch/1 -> Out1/1
  Constant28/1 -> Switch/2
  Constant1/1 -> Switch/1

== system ScriptDemo/Create/createMerge/After/SM6/SM6_Ki/Flow2Rpm/Subsystem1 ==
  In1 : Inport  OutDataTypeStr=int16
  Abs : Abs  OutDataTypeStr=single  SaturateOnIntegerOverflow=off
  Add6 : Sum  Inputs=+-  OutDataTypeStr=int16
  Compare To Constant : simulink/Logic and Bit Operations/Compare To Constant  relop=>=  const=0  OutDataTypeStr=boolean
  Compare To Constant1 : simulink/Logic and Bit Operations/Compare To Constant  relop=<=  const=10  OutDataTypeStr=boolean
  Constant6 : Constant  Value=0  OutDataTypeStr=uint16
  Constant7 : Constant  Value=10  OutDataTypeStr=uint16
  Logical Operator : Logic  AllPortsSameDT=off  OutDataTypeStr=boolean
  Switch : Switch  Criteria=u2 ~= 0  SaturateOnIntegerOverflow=off  InputSameDT=off
  Out1 : Outport
  wires:
  Add6/1 -> Switch/1
  Logical Operator/1 -> Switch/2
  Constant6/1 -> Switch/3
  Abs/1 -> Add6/2, Compare To Constant/1, Compare To Constant1/1
  Constant7/1 -> Add6/1
  Switch/1 -> Out1/1
  Compare To Constant1/1 -> Logical Operator/2
  Compare To Constant/1 -> Logical Operator/1
  In1/1 -> Abs/1

== system ScriptDemo/Create/createMerge/After/SM6/SM6_Ki/Flow2Rpm/Subsystem2 ==
  In1 : Inport  OutDataTypeStr=int16
  Abs : Abs  OutDataTypeStr=uint16  SaturateOnIntegerOverflow=off
  Add6 : Sum  Inputs=+-  OutDataTypeStr=int16
  Compare To Constant : simulink/Logic and Bit Operations/Compare To Constant  relop=>=  const=0  OutDataTypeStr=boolean
  Compare To Constant1 : simulink/Logic and Bit Operations/Compare To Constant  relop=<=  const=10  OutDataTypeStr=boolean
  Constant6 : Constant  Value=0  OutDataTypeStr=uint16
  Constant7 : Constant  Value=10  OutDataTypeStr=uint16
  Logical Operator : Logic  AllPortsSameDT=off  OutDataTypeStr=boolean
  Switch : Switch  Criteria=u2 ~= 0  SaturateOnIntegerOverflow=off  InputSameDT=off
  Out1 : Outport
  wires:
  Add6/1 -> Switch/1
  Logical Operator/1 -> Switch/2
  Constant6/1 -> Switch/3
  Abs/1 -> Add6/2, Compare To Constant/1, Compare To Constant1/1
  Constant7/1 -> Add6/1
  Switch/1 -> Out1/1
  Compare To Constant1/1 -> Logical Operator/2
  Compare To Constant/1 -> Logical Operator/1
  In1/1 -> Abs/1

== system ScriptDemo/Create/createMerge/After/SM6/SM6_Ki/Flow2Rpm/Subsystem3 ==
  In1 : Inport  OutDataTypeStr=int16
  Abs : Abs  OutDataTypeStr=uint16  SaturateOnIntegerOverflow=off
  Add6 : Sum  Inputs=+-  OutDataTypeStr=int16
  Compare To Constant : simulink/Logic and Bit Operations/Compare To Constant  relop=>=  const=0  OutDataTypeStr=boolean
  Compare To Constant1 : simulink/Logic and Bit Operations/Compare To Constant  relop=<=  const=10  OutDataTypeStr=boolean
  Constant6 : Constant  Value=0  OutDataTypeStr=uint16
  Constant7 : Constant  Value=10  OutDataTypeStr=uint16
  Logical Operator : Logic  AllPortsSameDT=off  OutDataTypeStr=boolean
  Switch : Switch  Criteria=u2 ~= 0  SaturateOnIntegerOverflow=off  InputSameDT=off
  Out1 : Outport
  wires:
  Add6/1 -> Switch/1
  Logical Operator/1 -> Switch/2
  Constant6/1 -> Switch/3
  Abs/1 -> Add6/2, Compare To Constant/1, Compare To Constant1/1
  Constant7/1 -> Add6/1
  Switch/1 -> Out1/1
  Compare To Constant1/1 -> Logical Operator/2
  Compare To Constant/1 -> Logical Operator/1
  In1/1 -> Abs/1

== system ScriptDemo/Create/createMerge/After/SM6/SM6_Ki/Flow2Rpm/Subsystem4 ==
  In1 : Inport  OutDataTypeStr=int16
  Abs : Abs  OutDataTypeStr=uint16  SaturateOnIntegerOverflow=off
  Add6 : Sum  Inputs=+-  OutDataTypeStr=int16
  Compare To Constant : simulink/Logic and Bit Operations/Compare To Constant  relop=>=  const=0  OutDataTypeStr=boolean
  Compare To Constant1 : simulink/Logic and Bit Operations/Compare To Constant  relop=<=  const=10  OutDataTypeStr=boolean
  Constant6 : Constant  Value=0  OutDataTypeStr=uint16
  Constant7 : Constant  Value=10  OutDataTypeStr=uint16
  Logical Operator : Logic  AllPortsSameDT=off  OutDataTypeStr=boolean
  Switch : Switch  Criteria=u2 ~= 0  SaturateOnIntegerOverflow=off  InputSameDT=off
  Out1 : Outport
  wires:
  Add6/1 -> Switch/1
  Logical Operator/1 -> Switch/2
  Constant6/1 -> Switch/3
  Abs/1 -> Add6/2, Compare To Constant/1, Compare To Constant1/1
  Constant7/1 -> Add6/1
  Switch/1 -> Out1/1
  Compare To Constant1/1 -> Logical Operator/2
  Compare To Constant/1 -> Logical Operator/1
  In1/1 -> Abs/1

== system ScriptDemo/Create/createMerge/After/SM6/SM6_Ki/Flow2Rpm/Subsystem5 ==
  In1 : Inport  OutDataTypeStr=int16
  Abs : Abs  OutDataTypeStr=uint16  SaturateOnIntegerOverflow=off
  Add6 : Sum  Inputs=+-  OutDataTypeStr=int16
  Compare To Constant : simulink/Logic and Bit Operations/Compare To Constant  relop=>=  const=0  OutDataTypeStr=boolean
  Compare To Constant1 : simulink/Logic and Bit Operations/Compare To Constant  relop=<=  const=10  OutDataTypeStr=boolean
  Constant6 : Constant  Value=0  OutDataTypeStr=uint16
  Constant7 : Constant  Value=10  OutDataTypeStr=uint16
  Logical Operator : Logic  AllPortsSameDT=off  OutDataTypeStr=boolean
  Switch : Switch  Criteria=u2 ~= 0  SaturateOnIntegerOverflow=off  InputSameDT=off
  Out1 : Outport
  wires:
  Add6/1 -> Switch/1
  Logical Operator/1 -> Switch/2
  Constant6/1 -> Switch/3
  Abs/1 -> Add6/2, Compare To Constant/1, Compare To Constant1/1
  Constant7/1 -> Add6/1
  Switch/1 -> Out1/1
  Compare To Constant1/1 -> Logical Operator/2
  Compare To Constant/1 -> Logical Operator/1
  In1/1 -> Abs/1

== system ScriptDemo/Create/createMerge/After/SM6/SM6_Ki/Flow2Rpm/XCP ==
  md_u8Blw : Inport
  Constant1 : Constant  Value=BlwHeatLevel_db
      settings: AttributesFormatString=%<Value>
  Constant28 : Constant  Value=BlwHeatLevel_sw
      settings: AttributesFormatString=%<Value>
  Switch : Switch  Criteria=u2 ~= 0  SaturateOnIntegerOverflow=off  InputSameDT=off
  Out1 : Outport
  wires:
  md_u8Blw/1 -> Switch/3
  Switch/1 -> Out1/1
  Constant28/1 -> Switch/2
  Constant1/1 -> Switch/1

== system ScriptDemo/Create/createMerge/After/SM6/SM6_Kp/Flow2Rpm/Subsystem1 ==
  In1 : Inport  OutDataTypeStr=int16
  Abs : Abs  OutDataTypeStr=single  SaturateOnIntegerOverflow=off
  Add6 : Sum  Inputs=+-  OutDataTypeStr=int16
  Compare To Constant : simulink/Logic and Bit Operations/Compare To Constant  relop=>=  const=0  OutDataTypeStr=boolean
  Compare To Constant1 : simulink/Logic and Bit Operations/Compare To Constant  relop=<=  const=10  OutDataTypeStr=boolean
  Constant6 : Constant  Value=0  OutDataTypeStr=uint16
  Constant7 : Constant  Value=10  OutDataTypeStr=uint16
  Logical Operator : Logic  AllPortsSameDT=off  OutDataTypeStr=boolean
  Switch : Switch  Criteria=u2 ~= 0  SaturateOnIntegerOverflow=off  InputSameDT=off
  Out1 : Outport
  wires:
  Add6/1 -> Switch/1
  Logical Operator/1 -> Switch/2
  Constant6/1 -> Switch/3
  Abs/1 -> Add6/2, Compare To Constant/1, Compare To Constant1/1
  Constant7/1 -> Add6/1
  Switch/1 -> Out1/1
  Compare To Constant1/1 -> Logical Operator/2
  Compare To Constant/1 -> Logical Operator/1
  In1/1 -> Abs/1

== system ScriptDemo/Create/createMerge/After/SM6/SM6_Kp/Flow2Rpm/Subsystem2 ==
  In1 : Inport  OutDataTypeStr=int16
  Abs : Abs  OutDataTypeStr=uint16  SaturateOnIntegerOverflow=off
  Add6 : Sum  Inputs=+-  OutDataTypeStr=int16
  Compare To Constant : simulink/Logic and Bit Operations/Compare To Constant  relop=>=  const=0  OutDataTypeStr=boolean
  Compare To Constant1 : simulink/Logic and Bit Operations/Compare To Constant  relop=<=  const=10  OutDataTypeStr=boolean
  Constant6 : Constant  Value=0  OutDataTypeStr=uint16
  Constant7 : Constant  Value=10  OutDataTypeStr=uint16
  Logical Operator : Logic  AllPortsSameDT=off  OutDataTypeStr=boolean
  Switch : Switch  Criteria=u2 ~= 0  SaturateOnIntegerOverflow=off  InputSameDT=off
  Out1 : Outport
  wires:
  Add6/1 -> Switch/1
  Logical Operator/1 -> Switch/2
  Constant6/1 -> Switch/3
  Abs/1 -> Add6/2, Compare To Constant/1, Compare To Constant1/1
  Constant7/1 -> Add6/1
  Switch/1 -> Out1/1
  Compare To Constant1/1 -> Logical Operator/2
  Compare To Constant/1 -> Logical Operator/1
  In1/1 -> Abs/1

== system ScriptDemo/Create/createMerge/After/SM6/SM6_Kp/Flow2Rpm/Subsystem3 ==
  In1 : Inport  OutDataTypeStr=int16
  Abs : Abs  OutDataTypeStr=uint16  SaturateOnIntegerOverflow=off
  Add6 : Sum  Inputs=+-  OutDataTypeStr=int16
  Compare To Constant : simulink/Logic and Bit Operations/Compare To Constant  relop=>=  const=0  OutDataTypeStr=boolean
  Compare To Constant1 : simulink/Logic and Bit Operations/Compare To Constant  relop=<=  const=10  OutDataTypeStr=boolean
  Constant6 : Constant  Value=0  OutDataTypeStr=uint16
  Constant7 : Constant  Value=10  OutDataTypeStr=uint16
  Logical Operator : Logic  AllPortsSameDT=off  OutDataTypeStr=boolean
  Switch : Switch  Criteria=u2 ~= 0  SaturateOnIntegerOverflow=off  InputSameDT=off
  Out1 : Outport
  wires:
  Add6/1 -> Switch/1
  Logical Operator/1 -> Switch/2
  Constant6/1 -> Switch/3
  Abs/1 -> Add6/2, Compare To Constant/1, Compare To Constant1/1
  Constant7/1 -> Add6/1
  Switch/1 -> Out1/1
  Compare To Constant1/1 -> Logical Operator/2
  Compare To Constant/1 -> Logical Operator/1
  In1/1 -> Abs/1
